simulink model "RefModel_AHRS"  (R2020b)
settings: Solver=ode1  StartTime=0.0  StopTime=10.0  FixedStep=Ts_Navi.Ts_Base  RelTol=1e-3
undefined symbols (not defined in the file or in its folder): compass_magDeclinationd, compass_pitchd, compass_rolld, compass_yawd
libraries: mspfiltlib x1, aerolibobsolete x1
settings Model: Creator=computer  LastModifiedBy=sl

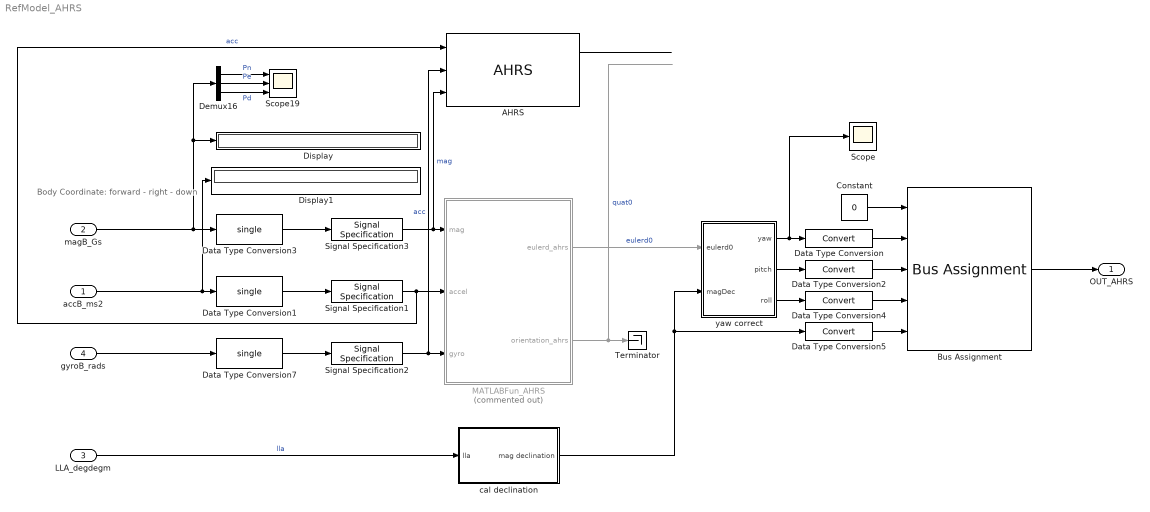
== system RefModel_AHRS ==
  note: Body Coordinate: forward - right - down
  accB_ms2 : Inport  PortDimensions=[1,3]
  magB_Gs : Inport  Port=2  PortDimensions=[1,3]
  LLA_degdegm : Inport  Port=3  PortDimensions=[1,3]
  gyroB_rads : Inport  Port=4  PortDimensions=[1,3]
  AHRS : mspfiltlib/AHRS  DispRefFrame=NED  DecimationFactor=1  InitialProcessNoise=ahrsfilter.defaultProcessNoise  OrientationFormat=quaternion  SimulateUsing=Interpreted execution  AccelerometerNoise=0.0001924722  GyroscopeNoise=9.1385e-5  MagnetometerNoise=0.1  GyroscopeDriftNoise=3.0462e-13  LinearAccelerationNoise=0.0096236100000000012  MagneticDisturbanceNoise=0.5  LinearAccelerationDecayFactor=0.5  MagneticDisturbanceDecayFactor=0.5  ExpectedMagneticFieldStrength=50
      settings: SourceProductBaseCode=TF,NV
  Bus Assignment : BusAssignment  AssignedSignals=compass_yawd,compass_pitchd,compass_rolld,compass_magDeclinationd
  Constant : Constant  Value=0  OutDataTypeStr=Bus: BUS_NAVI_ECOMPASS
  Data Type Conversion{,2,4..5} (4 alike) : DataTypeConversion
  Data Type Conversion1 : DataTypeConversion  OutDataTypeStr=single
  Data Type Conversion3 : DataTypeConversion  OutDataTypeStr=single
  Data Type Conversion7 : DataTypeConversion  OutDataTypeStr=single
  Demux16 : Demux  Outputs=3
  Display : Display
  Display1 : Display
  MATLABFun_AHRS : MATLAB Function  Commented=on  TreatAsAtomicUnit=on
  Scope : Scope
  Scope19 : Scope  NumInputPorts=3
  Signal Specification1 : SignalSpecification  Dimensions=[1,3]
  Signal Specification2 : SignalSpecification  Dimensions=[1,3]
  Signal Specification3 : SignalSpecification  Dimensions=[1,3]
  Terminator : Terminator
  cal declination : Subsystem
  yaw correct : Subsystem
  OUT_AHRS : Outport  OutDataTypeStr=Bus: BUS_NAVI_ECOMPASS
  wires:
  Data Type Conversion2/1 -> Bus Assignment/3
  Data Type Conversion3/1 -> Signal Specification3/1
  Demux16/1 -> Scope19/1  "Pn"
  Data Type Conversion5/1 -> Bus Assignment/5
  Signal Specification3/1 -> AHRS/3, MATLABFun_AHRS/1(mag)  "mag"
  yaw correct/2(pitch) -> Data Type Conversion2/1
  Demux16/2 -> Scope19/2  "Pe"
  Data Type Conversion4/1 -> Bus Assignment/4
  Signal Specification1/1 -> AHRS/1, MATLABFun_AHRS/2(accel)  "acc"
  cal declination/1(mag declination) -> Data Type Conversion5/1, yaw correct/2(magDec)
  yaw correct/1(yaw) -> Data Type Conversion/1, Scope/1
  yaw correct/3(roll) -> Data Type Conversion4/1
  MATLABFun_AHRS/2(orientation_ahrs) -> Terminator/1  "quat0"
  Data Type Conversion/1 -> Bus Assignment/2
  LLA_degdegm/1 -> cal declination/1(lla)  "lla"
  Data Type Conversion1/1 -> Signal Specification1/1
  MATLABFun_AHRS/1(eulerd_ahrs) -> yaw correct/1(eulerd0)  "eulerd0"
  accB_ms2/1 -> Display1/1, Data Type Conversion1/1
  magB_Gs/1 -> Demux16/1, Display/1, Data Type Conversion3/1
  Demux16/3 -> Scope19/3  "Pd"
  Data Type Conversion7/1 -> Signal Specification2/1
  gyroB_rads/1 -> Data Type Conversion7/1
  Signal Specification2/1 -> AHRS/2, MATLABFun_AHRS/3(gyro)  "acc"
  AHRS/1 -> ?
  Constant/1 -> Bus Assignment/1
  Bus Assignment/1 -> OUT_AHRS/1

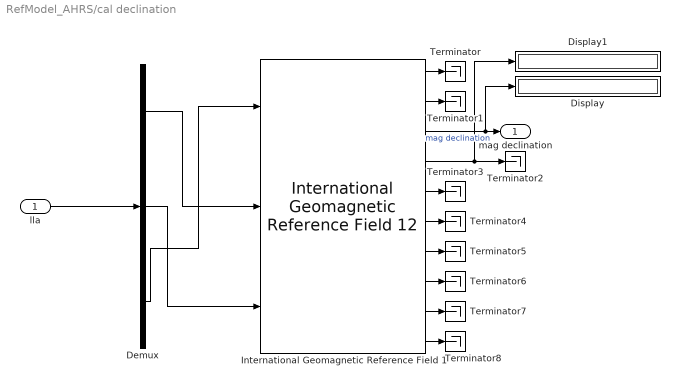
== system RefModel_AHRS/cal declination ==
  lla : Inport
  Demux : Demux  Outputs=3
  Display : Display
  Display1 : Display
  International Geomagnetic Reference Field 1 : aerolibobsolete/International Geomagnetic Reference Field 12  units=Metric (MKS)  time_in=off  month=January  day=1  year=2020  action=None  sv_out=on
      settings: SourceProductBaseCode=AE
  Terminator{,1..8} (9 alike) : Terminator
  mag declination : Outport
  wires:
  Demux/3 -> International Geomagnetic Reference Field 1/1
  Demux/1 -> International Geomagnetic Reference Field 1/2
  International Geomagnetic Reference Field 1/9 -> Terminator7/1
  International Geomagnetic Reference Field 1/10 -> Terminator8/1
  International Geomagnetic Reference Field 1/4 -> Display1/1, Terminator2/1
  International Geomagnetic Reference Field 1/1 -> Terminator/1
  Demux/2 -> International Geomagnetic Reference Field 1/3
  International Geomagnetic Reference Field 1/2 -> Terminator1/1
  International Geomagnetic Reference Field 1/3 -> Display/1, mag declination/1  "mag declination"
  International Geomagnetic Reference Field 1/5 -> Terminator3/1
  International Geomagnetic Reference Field 1/6 -> Terminator4/1
  International Geomagnetic Reference Field 1/8 -> Terminator6/1
  International Geomagnetic Reference Field 1/7 -> Terminator5/1
  lla/1 -> Demux/1

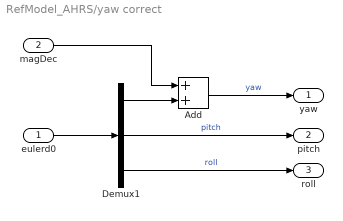
== system RefModel_AHRS/yaw correct ==
  eulerd0 : Inport
  magDec : Inport  Port=2
  Add : Sum
  Demux1 : Demux  Outputs=3
  yaw : Outport
  pitch : Outport  Port=2
  roll : Outport  Port=3
  wires:
  magDec/1 -> Add/1
  eulerd0/1 -> Demux1/1
  Demux1/2 -> pitch/1  "pitch"
  Demux1/3 -> roll/1  "roll"
  Demux1/1 -> Add/2
  Add/1 -> yaw/1  "yaw"

== matlab function RefModel_AHRS/MATLABFun_AHRS ==
  data: mag input; accel input; eulerd_ahrs output; orientation_ahrs output; gyro input
function [eulerd_ahrs,orientation_ahrs] = ahrs(mag,accel, gyro)
persistent filter_ahrs
if isempty(filter_ahrs)
    % AHRS
    filter_ahrs = ahrsfilter;
    filter_ahrs.SampleRate = 1000/12;
    filter_ahrs.AccelerometerNoise = 1e1*(3e-1).^2;
    filter_ahrs.GyroscopeNoise = 1e-2*(0.9e-1*pi/180).^2;
    filter_ahrs.MagnetometerNoise = (.5).^2; %
    filter_ahrs.LinearAccelerationDecayFactor = 0.9;   
    filter_ahrs.MagneticDisturbanceDecayFactor = 0.1;   
    filter_ahrs.ExpectedMagneticFieldStrength = 54;

end
%% AHRS
orientation_ahrs = compact(filter_ahrs(double(accel),double(gyro),double(mag)));
eulerd_ahrs = double(eulerd(orientation_ahrs));
end


function eout = eulerd(quat)
% rotate 'ZYX'
qa = quat(1);
qb = quat(2);
qc = quat(3);
qd = quat(4);
the1 = single(1);
the2 = single(2);

tmp = qb.*qd.*the2 - qa.*qc.*the2;
if tmp > the1
    tmp = the1;
elseif tmp < -the1
    tmp = -the1;
end
% tmp(tmp > the1) = the1;
% tmp(tmp < -the1) = -the1;
b = -asin(tmp);
a = atan2((qa.*qd.*the2 + qb.*qc.*the2),(qa.^2.*the2 - the1 + qb.^2.*the2));
c = atan2((qa.*qb.*the2 + qc.*qd.*the2),(qa.^2.*the2 - the1 + qd.^2.*the2));
eout = [a b c]*180/pi;
end

%
% function [eulerd0,quat0] = compass(i,accel,mag,imuUpdateFs,magUpdateFs)
%     fs = imuUpdateFs;
%     quat0 = zeros(1,4);
%     eulerd0 = zeros(1,3);
%     if rem(i,fs/magUpdateFs) == 0 && i ~= 1
%         quat0 = compact(ecompass(accel,mag));
%         eulerd0 = eulerd(quat0);
%     end
% end
